simulink model "std_d_func"  (R2022b)
settings: Solver=FixedStepAuto  StartTime=0.0  StopTime=Ts*1000  FixedStep=Ts  RelTol=1e-3
values from neighbouring files (symbols this model uses):
  Ak = [1 Ts Ts^2/2;0 1 Ts;0 0 1]    [para.m]
  Bk = [0;0;0]    [para.m]
  Ck = [1 0 0]    [para.m]
  Dk = 0    [para.m]
  P0 = [10 0 0; 0 10 0;0 0 10]    [para.m]
  Qk = [0;0;0]    [para.m]
  Rk = 30^2    (= 900)    [para.m]
  Ts = 5    [para.m]
  x0_est = [0;0;0]    [para.m]
  x0_init = [0;0;0]    [para.m]
libraries: simulink x2
settings Model: Creator=mxiaoxin  LastModifiedBy=mxiaoxin

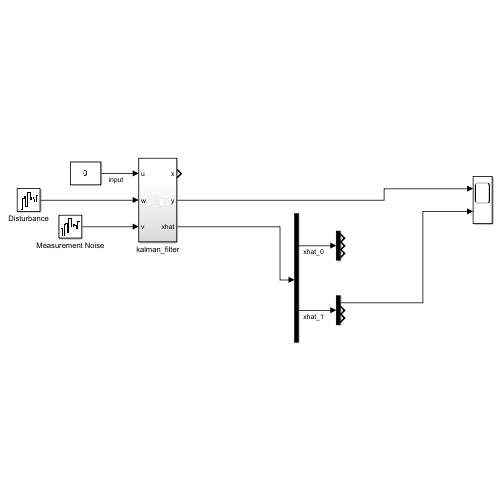
[thumbnail: Simulink's stored preview of the top-level diagram]
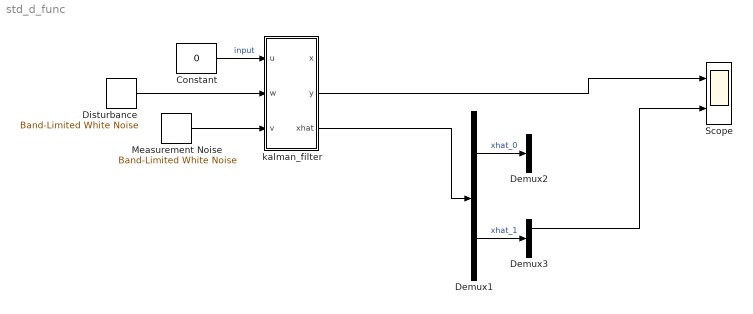
== system std_d_func ==
  Constant : Constant  Value=0
  Demux1 : Demux  Outputs=2
  Demux2 : Demux  Outputs=3
  Demux3 : Demux  Outputs=3
  Disturbance : simulink/Sources/Band-Limited White Noise  Cov=Qk  Ts=Ts  seed=[23341]
  Measurement Noise : simulink/Sources/Band-Limited White Noise  Cov=Rk  Ts=Ts  seed=13412
  Scope : Scope  NumInputPorts=2
  kalman_filter : Subsystem
  wires:
  kalman_filter/3(xhat) -> Demux1/1
  Demux1/2 -> Demux3/1  "xhat_1"
  kalman_filter/2(y) -> Scope/1
  Demux1/1 -> Demux2/1  "xhat_0"
  Disturbance/1 -> kalman_filter/2(w)
  Measurement Noise/1 -> kalman_filter/3(v)
  Demux3/1 -> Scope/2
  Constant/1 -> kalman_filter/1(u)  "input"

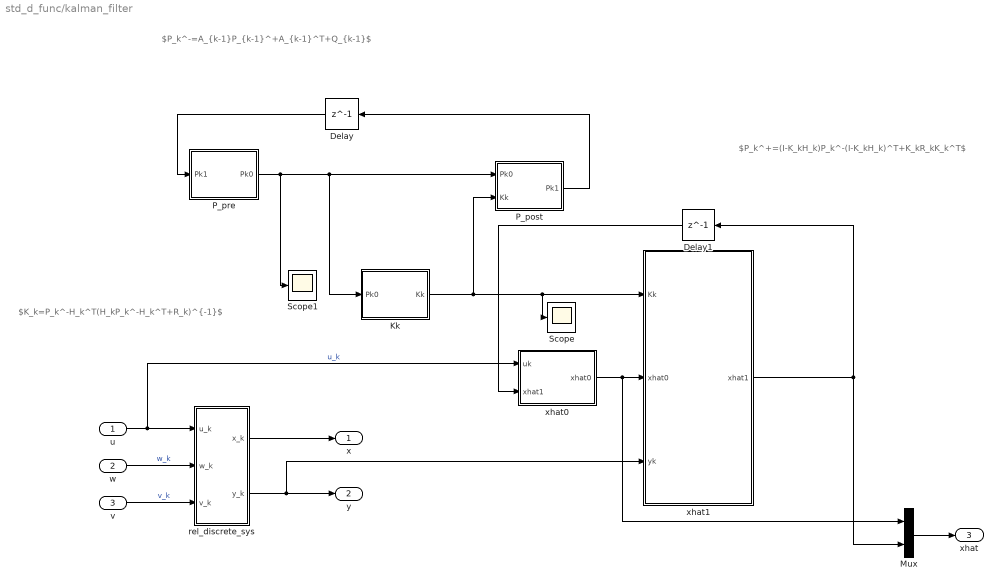
== system std_d_func/kalman_filter ==
  note: $P_k^+=(I-K_kH_k)P_k^-(I-K_kH_k)^T+K_kR_kK_k^T$
  note: $K_k=P_k^-H_k^T(H_kP_k^-H_k^T+R_k)^{-1}$
  note: $P_k^-=A_{k-1}P_{k-1}^+A_{k-1}^T+Q_{k-1}$
  u : Inport
  w : Inport  Port=2
  v : Inport  Port=3
  Delay : Delay  DelayLength=1  InitialCondition=P0
  Delay1 : Delay  DelayLength=1  InitialCondition=x0_est
  Kk : MATLAB Function  TreatAsAtomicUnit=on
  Mux : Mux  Inputs=2
  P_post : MATLAB Function  TreatAsAtomicUnit=on
  P_pre : MATLAB Function  TreatAsAtomicUnit=on
  Scope : Scope
  Scope1 : Scope
  rel_discrete_sys : Subsystem
  xhat0 : MATLAB Function  TreatAsAtomicUnit=on
  xhat1 : MATLAB Function  TreatAsAtomicUnit=on
  x : Outport
  y : Outport  Port=2
  xhat : Outport  Port=3
  wires:
  u/1 -> xhat0/1(uk), rel_discrete_sys/1(u_k)  "u_k"
  w/1 -> rel_discrete_sys/2(w_k)  "w_k"
  v/1 -> rel_discrete_sys/3(v_k)  "v_k"
  rel_discrete_sys/1(x_k) -> x/1
  xhat0/1(xhat0) -> Mux/1, xhat1/2(xhat0)
  rel_discrete_sys/2(y_k) -> xhat1/3(yk), y/1
  Kk/1(Kk) -> P_post/2(Kk), Scope/1, xhat1/1(Kk)
  Delay/1 -> P_pre/1(Pk1)
  xhat1/1(xhat1) -> Delay1/1, Mux/2
  Delay1/1 -> xhat0/2(xhat1)
  Mux/1 -> xhat/1
  P_post/1(Pk1) -> Delay/1
  P_pre/1(Pk0) -> Scope1/1, Kk/1(Pk0), P_post/1(Pk0)

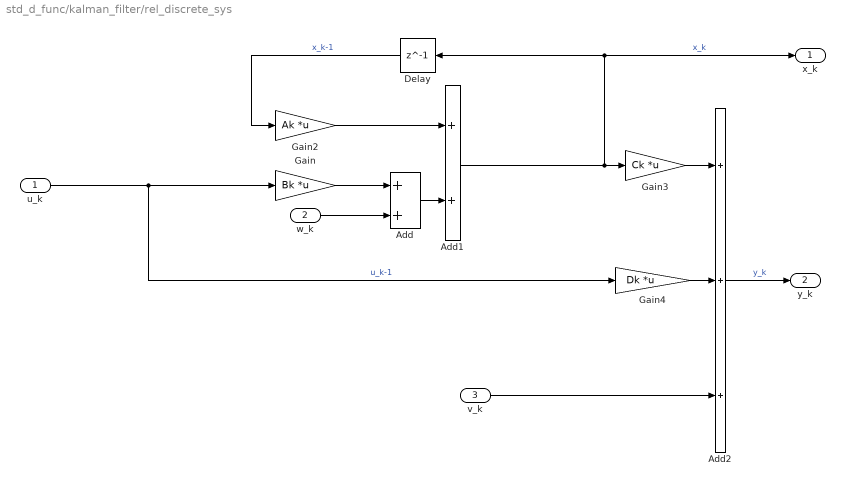
== system std_d_func/kalman_filter/rel_discrete_sys ==
  u_k : Inport
  w_k : Inport  Port=2
  v_k : Inport  Port=3
  Add : Sum
  Add1 : Sum
  Add2 : Sum  Inputs=+++
  Delay : Delay  DelayLength=1  InitialCondition=x0_init
  Gain : Gain  Gain=Bk  Multiplication=Matrix(K*u)
  Gain2 : Gain  Gain=Ak  Multiplication=Matrix(K*u)
  Gain3 : Gain  Gain=Ck  Multiplication=Matrix(K*u)
  Gain4 : Gain  Gain=Dk  Multiplication=Matrix(K*u)
  x_k : Outport
  y_k : Outport  Port=2
  wires:
  Delay/1 -> Gain2/1  "x_k-1"
  Gain4/1 -> Add2/2
  Add1/1 -> Gain3/1, x_k/1, Delay/1  "x_k"
  v_k/1 -> Add2/3
  u_k/1 -> Gain/1, Gain4/1  "u_k-1"
  Gain2/1 -> Add1/1
  Gain3/1 -> Add2/1
  w_k/1 -> Add/2
  Add2/1 -> y_k/1  "y_k"
  Add/1 -> Add1/2
  Gain/1 -> Add/1

== matlab function std_d_func/kalman_filter/P_post ==
  data: Pk0 input; Pk1 output; Kk input; Ck parameter; Rk parameter
function Pk1 = fcn(Pk0,Kk, Ck, Rk)

Pk1=(eye(size(Kk*Ck,1))-Kk*Ck)*Pk0*(eye(size(Kk*Ck,1))-Kk*Ck)'+Kk*Rk*Kk';

== matlab function std_d_func/kalman_filter/P_pre ==
  data: Pk0 output; Pk1 input; Ak parameter; Qk parameter
function Pk0 = fcn(Pk1,Ak,Qk)

Pk0 = Ak*Pk1*Ak'+Qk;

== matlab function std_d_func/kalman_filter/Kk ==
  data: Pk0 input; Kk output; Ck parameter; Rk parameter
function Kk = fcn(Pk0,Ck, Rk)

Kk = Pk0*Ck'/(Ck*Pk0*Ck'+Rk);

== matlab function std_d_func/kalman_filter/xhat1 ==
  data: Kk input; xhat0 input; xhat1 output; yk input; Ck parameter
function xhat1 = fcn(Kk,xhat0,yk,Ck)

xhat1 = xhat0+Kk*(yk-Ck*xhat0);

== matlab function std_d_func/kalman_filter/xhat0 ==
  data: uk input; xhat0 output; xhat1 input; Ak parameter; Bk parameter
function xhat0 = fcn(uk,xhat1,Ak, Bk)

xhat0 = Ak*xhat1+Bk*uk;
